simulink model "Plant_inversion_nominal"  (R2019b)
settings: Solver=ode3  StartTime=-12  StopTime=15.0  FixedStep=0.001  RelTol=1e-3
settings Model: Creator=Aurelio Piazzi  LastModifiedBy=Aurus

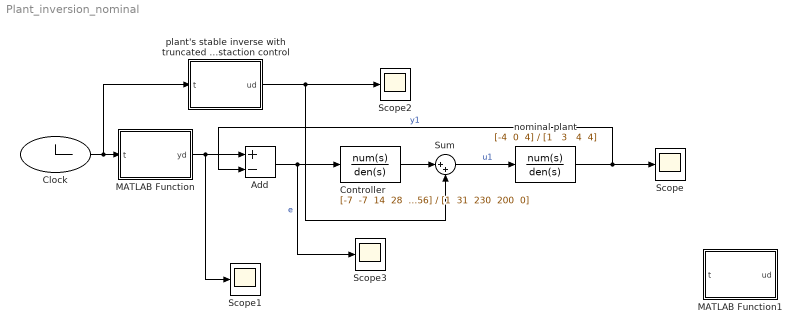
== system Plant_inversion_nominal ==
  Add : Sum  Inputs=+-
  Clock : Clock
  Controller : TransferFcn  Numerator="[-7  -7  14  28  56]"  Denominator="[1  31  230  200  0]"
  MATLAB Function : MATLAB Function  TreatAsAtomicUnit=on
  MATLAB Function1 : MATLAB Function  TreatAsAtomicUnit=on
  Scope{,1..3} (4 alike) : Scope
  Sum : Sum  Inputs=|++
  nominal plant : TransferFcn  Numerator="[-4  0  4]"  Denominator="[1   3   4  4]"
  "plant's stable inverse with truncated postaction control " : MATLAB Function  TreatAsAtomicUnit=on
  wires:
  MATLAB Function/1(yd) -> Scope1/1, Add/1
  Add/1 -> Controller/1, Scope3/1  "e"
  nominal plant/1 -> Add/2, Scope/1  "y1"
  Clock/1 -> "plant's stable inverse with truncated postaction control "/1(t), MATLAB Function/1(t)
  Controller/1 -> Sum/1
  Sum/1 -> nominal plant/1  "u1"
  "plant's stable inverse with truncated postaction control "/1(ud) -> Scope2/1, Sum/2

== matlab function Plant_inversion_nominal/MATLAB Function1 ==
  data: t input; ud output
function ud = ud(t)
 if(t<0)
     ud = (1/3)*exp(t)+(5/3)*exp(t-3);
 elseif (t<3)
     ud = -(1/9)*t+(1/9)*t^2-(2/27)*t^3-(5/18)*exp(-t)+11/18+(5/3)*exp(t-3);
 else
     ud = 1-(5/18)*exp(-t)-(1/18)*exp(3-t);
 end

== matlab function Plant_inversion_nominal/MATLAB Function ==
  data: t input; yd output
function yd = yd(t)
 if(t<0)
     yd = 0;
 elseif (t<3)
     yd = (1/3)*t^2-(2/27)*t^3;
 else
     yd = 1;
 end

== matlab function Plant_inversion_nominal/plant's stable inverse with truncated postaction control  ==
  data: t input; ud output
function ud = ud(t)
 if(t<0)
     ud = (1/3)*exp(t)+(5/3)*exp(t-3);
 elseif (t<3)
     ud = -(1/9)*t+(1/9)*t^2-(2/27)*t^3-(5/18)*exp(-t)+11/18+(5/3)*exp(t-3);
 elseif (t < 3 + 6.97)
     ud = 1-(5/18)*exp(-t)-(1/18)*exp(3-t);
 else
     ud = 1;
 end
